simulink model "simu_control_robot_2"  (Simulink 7.9)
settings: Solver=ode3  StartTime=0.0  StopTime=3  FixedStep=0.01  RelTol=1e-3
values from neighbouring files (symbols this model uses):
  k1 = -q(1)*q(2)-1    [WPG_results.m]    (also in WPG_results_10.m; WPG_results_2.m; WPG_results_3.m; WPG_results_4.m)
  k2 = (q(1)+q(2))/-q(3)    [WPG_results.m]    (also in WPG_results_10.m; WPG_results_2.m; WPG_results_3.m; WPG_results_4.m)
  k3 = w    [WPG_results.m]    (also in WPG_results_10.m; WPG_results_2.m; WPG_results_3.m; WPG_results_4.m)
  sx_d = [time sx_d]    [WPG_results.m]    (also in WPG_sim.m; control_layer_zmp_com_init.m = [time sx_d_y]; control_layer_zmp_com_init_2.m = [time sx_d_x])
  w = wpg_param.w    [WPG_results.m]    (also in WPG_results_10.m; WPG_results_2.m; WPG_results_3.m; WPG_results_4.m)
  x_d = [time x_d]    [WPG_results.m]    (also in WPG_sim.m; control_layer_zmp_com_init.m = [time x_d_y]; control_layer_zmp_com_init_2.m = [time x_d_x])
undefined symbols (not defined in the file or in its folder): wpg_param
libraries: simulink x1
settings Model: Creator=pajon  LastModifiedBy=pajon

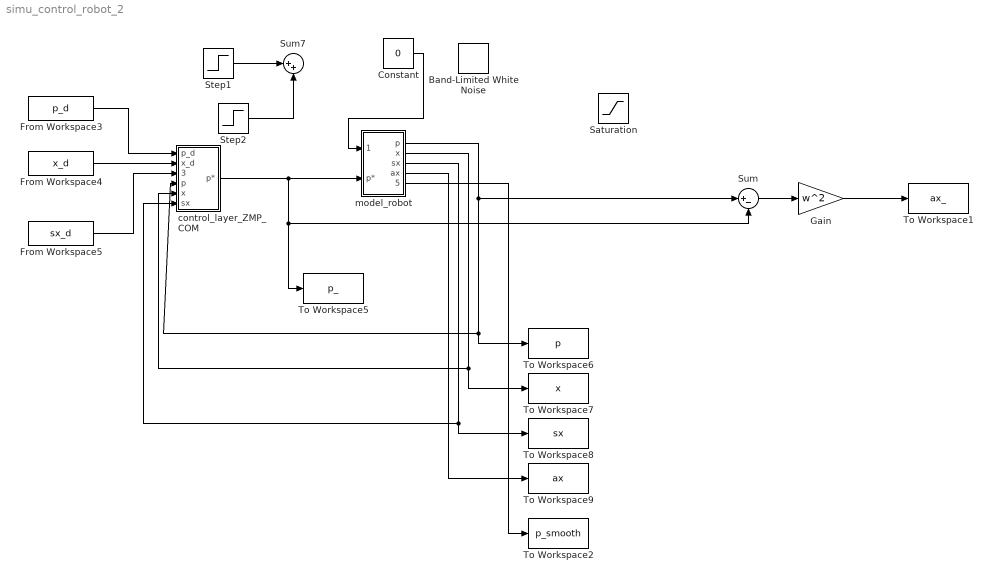
== system simu_control_robot_2 ==
  Band-Limited White Noise : simulink/Sources/Band-Limited White Noise  Cov=[0.000001]  Ts=0.01  seed=[23341]
  Constant : Constant  Value=0
  From Workspace3 : FromWorkspace  VariableName=p_d  SampleTime=0
  From Workspace4 : FromWorkspace  VariableName=x_d  SampleTime=0
  From Workspace5 : FromWorkspace  VariableName=sx_d  SampleTime=0
  Gain : Gain  Gain=w^2
  Saturation : Saturate  UpperLimit=wpg_param.fronttoankle  LowerLimit=-wpg_param.backtoankle
  Step1 : Step  Time=0.4  After=+10/wpg_param.m  SampleTime=0
  Step2 : Step  Time=1.5  After=-10/wpg_param.m  SampleTime=0
  Sum : Sum  Inputs=|+-
  Sum7 : Sum  Inputs=|++
  To Workspace1 : ToWorkspace  VariableName=ax_  SampleTime=-1
  To Workspace2 : ToWorkspace  VariableName=p_smooth  SampleTime=-1
  To Workspace5 : ToWorkspace  VariableName=p_  SampleTime=-1
  To Workspace6 : ToWorkspace  VariableName=p  SampleTime=-1
  To Workspace7 : ToWorkspace  VariableName=x  SampleTime=-1
  To Workspace8 : ToWorkspace  VariableName=sx  SampleTime=-1
  To Workspace9 : ToWorkspace  VariableName=ax  SampleTime=-1
  control_layer_ZMP_COM : Subsystem
  model_robot : Subsystem
  wires:
  From Workspace5/1 -> control_layer_ZMP_COM/3(sx_d)
  model_robot/1(p) -> To Workspace6/1, control_layer_ZMP_COM/4(p), Sum/1
  model_robot/2(x) -> To Workspace7/1, control_layer_ZMP_COM/5(x)
  model_robot/3(sx) -> To Workspace8/1, control_layer_ZMP_COM/6(sx)
  model_robot/4(ax) -> To Workspace9/1
  Sum/1 -> Gain/1
  Gain/1 -> To Workspace1/1
  control_layer_ZMP_COM/1(p*) -> model_robot/2(p*), To Workspace5/1, Sum/2
  From Workspace4/1 -> control_layer_ZMP_COM/2(x_d)
  Step1/1 -> Sum7/1
  Step2/1 -> Sum7/2
  From Workspace3/1 -> control_layer_ZMP_COM/1(p_d)
  Constant/1 -> model_robot/1(perturb)
  model_robot/5(p_smooth) -> To Workspace2/1

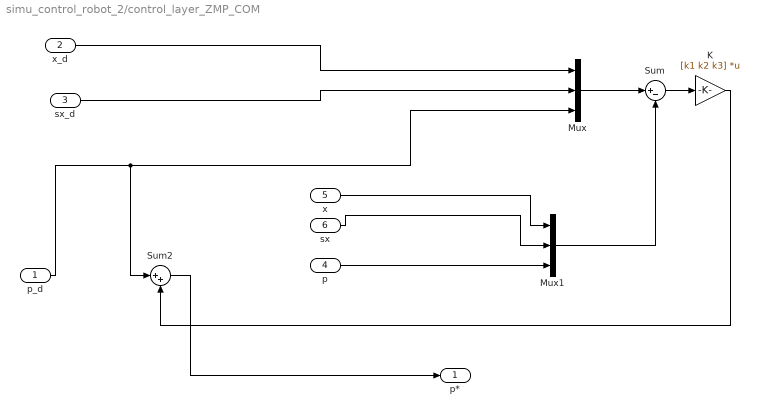
== system simu_control_robot_2/control_layer_ZMP_COM ==
  p_d : Inport
  x_d : Inport  Port=2
  sx_d : Inport  Port=3
  p : Inport  Port=4
  x : Inport  Port=5
  sx : Inport  Port=6
  K : Gain  Gain=[k1 k2 k3]  Multiplication=Matrix(K*u)
  Mux : Mux  Inputs=3
  Mux1 : Mux  Inputs=3
  Sum : Sum  Inputs=|+-
  Sum2 : Sum  Inputs=|++
  p* : Outport
  wires:
  Mux/1 -> Sum/1
  Mux1/1 -> Sum/2
  Sum/1 -> K/1
  K/1 -> Sum2/2
  Sum2/1 -> p*/1
  x/1 -> Mux1/1
  sx/1 -> Mux1/2
  p_d/1 -> Mux/3, Sum2/1
  x_d/1 -> Mux/1
  sx_d/1 -> Mux/2
  p/1 -> Mux1/3

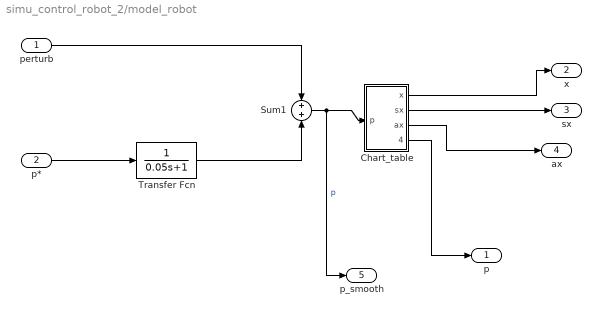
== system simu_control_robot_2/model_robot ==
  perturb : Inport
  p* : Inport  Port=2
  Chart_table : Subsystem
  Sum1 : Sum
  Transfer Fcn : TransferFcn  Denominator=[0.05 1]
  p : Outport
  x : Outport  Port=2
  sx : Outport  Port=3
  ax : Outport  Port=4
  p_smooth : Outport  Port=5
  wires:
  perturb/1 -> Sum1/1
  p*/1 -> Transfer Fcn/1
  Chart_table/1(x) -> x/1
  Chart_table/2(sx) -> sx/1
  Chart_table/3(ax) -> ax/1
  Transfer Fcn/1 -> Sum1/2
  Sum1/1 -> Chart_table/1(p), p_smooth/1  "p"
  Chart_table/4(p_real) -> p/1

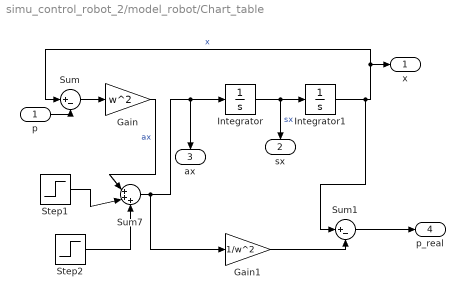
== system simu_control_robot_2/model_robot/Chart_table ==
  p : Inport
  Gain : Gain  Gain=w^2
  Gain1 : Gain  Gain=1/w^2
  Integrator : Integrator  InitialCondition=sx_d(1,2)
  Integrator1 : Integrator  InitialCondition=x_d(1,2)
  Step1 : Step  Time=0.4  After=+0/wpg_param.m  SampleTime=0
  Step2 : Step  Time=1.5  After=-0/wpg_param.m  SampleTime=0
  Sum : Sum  Inputs=|+-
  Sum1 : Sum  Inputs=|+-
  Sum7 : Sum  Inputs=|+++
  x : Outport
  sx : Outport  Port=2
  ax : Outport  Port=3
  p_real : Outport  Port=4
  wires:
  Integrator/1 -> Integrator1/1, sx/1  "sx"
  Integrator1/1 -> Sum/1, x/1, Sum1/1  "x"
  p/1 -> Sum/2
  Sum/1 -> Gain/1
  Gain/1 -> Sum7/1  "ax"
  Sum7/1 -> Integrator/1, ax/1, Gain1/1
  Sum1/1 -> p_real/1
  Gain1/1 -> Sum1/2
  Step1/1 -> Sum7/2
  Step2/1 -> Sum7/3
